simulink library "cables_lib"  (Simulink 7.8)
settings: Solver=ode45  StartTime=0.0  StopTime=10.0  RelTol=1e-3
libraries: powerlib x10
settings Model: Creator=RE25624  LastModifiedBy=g73labuser

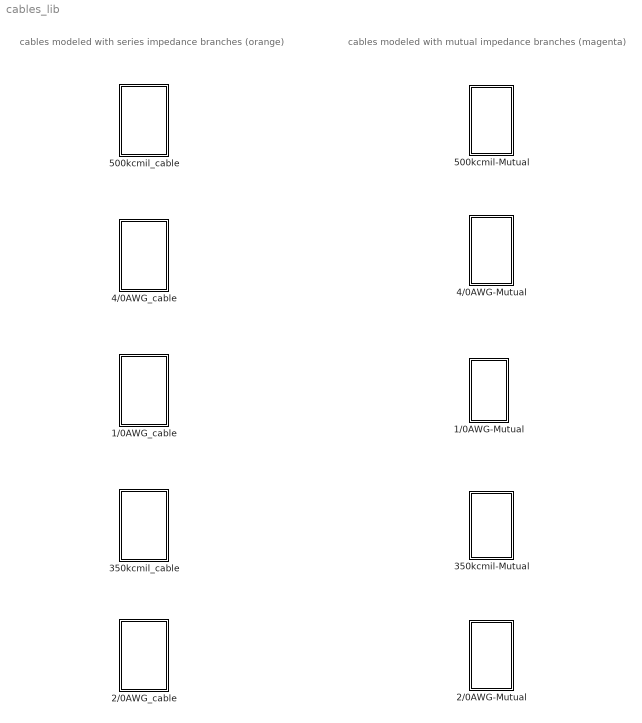
== system cables_lib ==
  note: cables modeled with mutual impedance branches (magenta)
  note: cables modeled with series impedance branches (orange)
  1/0AWG-Mutual : Subsystem  mask(1/0AWG cable){length=1, par_sets=1, ratio=3}
      mask prompts: length "Length [ft]"; par_sets "No. of parallel sets"; ratio "Z0 / Z1 Impedane Ratio"
      mask help:
      | This model approximates a cable using a mutual impedance branch.
      |
      | The parameter values for the positive sequence are based on IEEE 141-1993 Table 4A-7b.
      |
      | The zero-to-positive sequence (Z0/Z1) ratio permits the calculation of the mutual impedance.
      |
      | Example, for a effectively grounded system is in ranges Z0/Z1 < 3.
  1/0AWG_cable : Subsystem  mask(1/0AWG cable){length=50, par_sets=1}
      mask prompts: length "Length [ft]"; par_sets "No. of parallel sets"
      mask help:
      | This block represents a 1/0AWG cable based on Table 4A-7  60 Hz impedance data for three-phase copper cable circuits, in approximate ohms per ft at 75 degrees C (b) Three-conductor cable
      |
      | Page 181 of the Red Book
  2/0AWG-Mutual : Subsystem  mask(2/0AWG cable){length=1, par_sets=1, ratio=3}
      mask prompts: length "Length [ft]"; par_sets "No. of parallel sets"; ratio "Z0 / Z1 Impedane Ratio"
      mask help:
      | This model approximates a cable using a mutual impedance branch.
      |
      | The parameter values for the positive sequence are based on IEEE 141-1993 Table 4A-7b.
      |
      | The zero-to-positive sequence (Z0/Z1) ratio permits the calculation of the mutual impedance.
      |
      | Example, for a effectively grounded system is in ranges Z0/Z1 < 3.
  2/0AWG_cable : Subsystem  mask(2/0AWG cable){length=50, par_sets=1}
      mask prompts: length "Length [ft]"; par_sets "No. of parallel sets"
      mask help:
      | This block represents a 2/0AWG cable based on Table 4A-7  60 Hz impedance data for three-phase copper cable circuits, in approximate ohms per ft at 75 degrees C (b) Three-conductor cable
      |
      | Page 181 of the Red Book
  350kcmil-Mutual : Subsystem  mask(350kcmil cable){length=1, par_sets=1, ratio=3}
      mask prompts: length "Length [ft]"; par_sets "No. of parallel sets"; ratio "Z0 / Z1 Impedane Ratio"
      mask help:
      | This model approximates a cable using a mutual impedance branch.
      |
      | The parameter values for the positive sequence are based on IEEE 141-1993 Table 4A-7b.
      |
      | The zero-to-positive sequence (Z0/Z1) ratio permits the calculation of the mutual impedance.
      |
      | Example, for a effectively grounded system is in ranges Z0/Z1 < 3.
  350kcmil_cable : Subsystem  mask(350kcmil cable){length=50, par_sets=1}
      mask prompts: length "Length [ft]"; par_sets "No. of parallel sets"
      mask help:
      | This block represents a 350kcmil cable based on Table 4A-7  60 Hz impedance data for three-phase copper cable circuits, in approximate ohms per ft at 75 degrees C (b) Three-conductor cable
      |
      | Page 181 of the Red Book
  4/0AWG-Mutual : Subsystem  mask(4/0AWG cable){length=1, par_sets=1, ratio=3}
      mask prompts: length "Length [ft]"; par_sets "No. of parallel sets"; ratio "Z0 / Z1 Impedane Ratio"
      mask help:
      | This model approximates a cable using a mutual impedance branch.
      |
      | The parameter values for the positive sequence are based on IEEE 141-1993 Table 4A-7b.
      |
      | The zero-to-positive sequence (Z0/Z1) ratio permits the calculation of the mutual impedance.
      |
      | Example, for a effectively grounded system is in ranges Z0/Z1 < 3.
  4/0AWG_cable : Subsystem  mask(4/0AWG cable){length=50, par_sets=1}
      mask prompts: length "Length [ft]"; par_sets "No. of parallel sets"
      mask help:
      | This block represents a 4/0AWG cable based on Table 4A-7  60 Hz impedance data for three-phase copper cable circuits, in approximate ohms per ft at 75 degrees C (b) Three-conductor cable
      |
      | Page 181 of the Red Book
  500kcmil-Mutual : Subsystem  mask(500kcmil cable){length=1, par_sets=1, ratio=3}
      mask prompts: length "Length [ft]"; par_sets "No. of parallel sets"; ratio "Z0 / Z1 Impedane Ratio"
      mask help:
      | This model approximates a cable using a mutual impedance branch.
      |
      | The parameter values for the positive sequence are based on IEEE 141-1993 Table 4A-7b.
      |
      | The zero-to-positive sequence (Z0/Z1) ratio permits the calculation of the mutual impedance.
      |
      | Example, for a effectively grounded system is in ranges Z0/Z1 < 3.
  500kcmil_cable : Subsystem  mask(500kcmil cable){length=50, par_sets=1}
      mask prompts: length "Length [ft]"; par_sets "No. of parallel sets"
      mask help:
      | This block represents a 500kcmil cable based on Table 4A-7  60 Hz impedance data for three-phase copper cable circuits, in approximate ohms per ft at 75 degrees C (b) Three-conductor cable
      |
      | Page 181 of the Red Book

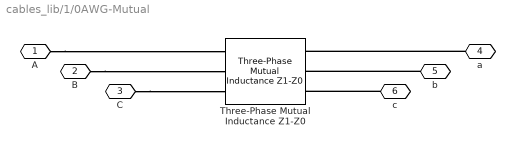
== system cables_lib/1/0AWG-Mutual ==
  Three-Phase Mutual Inductance Z1-Z0 : powerlib/Elements/Three-Phase Mutual Inductance Z1-Z0  LConnTagsString=a|b|c  RConnTagsString=A|B|C  PositiveSequence="[(0.000128*length/par_sets)  (1.0982e-007*length/par_sets)]"  ZeroSequence="[(0.000128*length/par_sets)  (1.0982e-007*length/par_sets)]*ratio"
  A : PMIOPort  Port=1  Side=Left
  B : PMIOPort  Port=2  Side=Left
  C : PMIOPort  Port=3  Side=Left
  a : PMIOPort  Port=4  Side=Right
  b : PMIOPort  Port=5  Side=Right
  c : PMIOPort  Port=6  Side=Right
  connections:
  c/RConn1 -- Three-Phase Mutual Inductance Z1-Z0/RConn3
  C/RConn1 -- Three-Phase Mutual Inductance Z1-Z0/LConn3
  b/RConn1 -- Three-Phase Mutual Inductance Z1-Z0/RConn2
  B/RConn1 -- Three-Phase Mutual Inductance Z1-Z0/LConn2
  a/RConn1 -- Three-Phase Mutual Inductance Z1-Z0/RConn1
  A/RConn1 -- Three-Phase Mutual Inductance Z1-Z0/LConn1

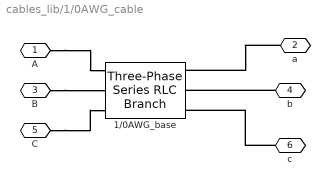
== system cables_lib/1/0AWG_cable ==
  1/0AWG_base : powerlib/Elements/Three-Phase Series RLC Branch  LConnTagsString=A|B|C  RConnTagsString=A|B|C  BranchType=RL  Resistance=0.000128*length/par_sets  Inductance=1.0982e-007*length/par_sets  Capacitance=0  Measurements=None
  A : PMIOPort  Port=1  Side=Left
  a : PMIOPort  Port=2  Side=Right
  B : PMIOPort  Port=3  Side=Left
  b : PMIOPort  Port=4  Side=Right
  C : PMIOPort  Port=5  Side=Left
  c : PMIOPort  Port=6  Side=Right
  connections:
  A/RConn1 -- 1/0AWG_base/LConn1
  a/RConn1 -- 1/0AWG_base/RConn1
  B/RConn1 -- 1/0AWG_base/LConn2
  b/RConn1 -- 1/0AWG_base/RConn2
  C/RConn1 -- 1/0AWG_base/LConn3
  c/RConn1 -- 1/0AWG_base/RConn3

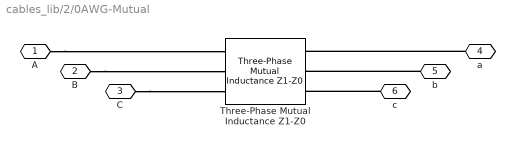
== system cables_lib/2/0AWG-Mutual ==
  Three-Phase Mutual Inductance Z1-Z0 : powerlib/Elements/Three-Phase Mutual Inductance Z1-Z0  LConnTagsString=a|b|c  RConnTagsString=A|B|C  PositiveSequence="[(0.000102*length/par_sets)  (1.0796e-007*length/par_sets)]"  ZeroSequence="[(0.000102*length/par_sets)  (1.0796e-007*length/par_sets)]*ratio"
  A : PMIOPort  Port=1  Side=Left
  B : PMIOPort  Port=2  Side=Left
  C : PMIOPort  Port=3  Side=Left
  a : PMIOPort  Port=4  Side=Right
  b : PMIOPort  Port=5  Side=Right
  c : PMIOPort  Port=6  Side=Right
  connections:
  c/RConn1 -- Three-Phase Mutual Inductance Z1-Z0/RConn3
  C/RConn1 -- Three-Phase Mutual Inductance Z1-Z0/LConn3
  b/RConn1 -- Three-Phase Mutual Inductance Z1-Z0/RConn2
  B/RConn1 -- Three-Phase Mutual Inductance Z1-Z0/LConn2
  a/RConn1 -- Three-Phase Mutual Inductance Z1-Z0/RConn1
  A/RConn1 -- Three-Phase Mutual Inductance Z1-Z0/LConn1

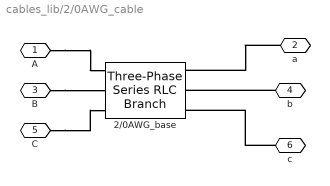
== system cables_lib/2/0AWG_cable ==
  2/0AWG_base : powerlib/Elements/Three-Phase Series RLC Branch  LConnTagsString=A|B|C  RConnTagsString=A|B|C  BranchType=RL  Resistance=0.000102*length/par_sets  Inductance=1.0796e-007*length/par_sets  Capacitance=0  Measurements=None
  A : PMIOPort  Port=1  Side=Left
  a : PMIOPort  Port=2  Side=Right
  B : PMIOPort  Port=3  Side=Left
  b : PMIOPort  Port=4  Side=Right
  C : PMIOPort  Port=5  Side=Left
  c : PMIOPort  Port=6  Side=Right
  connections:
  A/RConn1 -- 2/0AWG_base/LConn1
  a/RConn1 -- 2/0AWG_base/RConn1
  B/RConn1 -- 2/0AWG_base/LConn2
  b/RConn1 -- 2/0AWG_base/RConn2
  C/RConn1 -- 2/0AWG_base/LConn3
  c/RConn1 -- 2/0AWG_base/RConn3

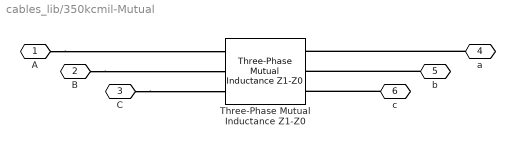
== system cables_lib/350kcmil-Mutual ==
  Three-Phase Mutual Inductance Z1-Z0 : powerlib/Elements/Three-Phase Mutual Inductance Z1-Z0  LConnTagsString=a|b|c  RConnTagsString=A|B|C  PositiveSequence="[(3.78e-005*length/par_sets)  (9.8941e-008*length/par_sets)]"  ZeroSequence="[(3.78e-005*length/par_sets)  (9.8941e-008*length/par_sets)]*ratio"
  A : PMIOPort  Port=1  Side=Left
  B : PMIOPort  Port=2  Side=Left
  C : PMIOPort  Port=3  Side=Left
  a : PMIOPort  Port=4  Side=Right
  b : PMIOPort  Port=5  Side=Right
  c : PMIOPort  Port=6  Side=Right
  connections:
  c/RConn1 -- Three-Phase Mutual Inductance Z1-Z0/RConn3
  C/RConn1 -- Three-Phase Mutual Inductance Z1-Z0/LConn3
  b/RConn1 -- Three-Phase Mutual Inductance Z1-Z0/RConn2
  B/RConn1 -- Three-Phase Mutual Inductance Z1-Z0/LConn2
  a/RConn1 -- Three-Phase Mutual Inductance Z1-Z0/RConn1
  A/RConn1 -- Three-Phase Mutual Inductance Z1-Z0/LConn1

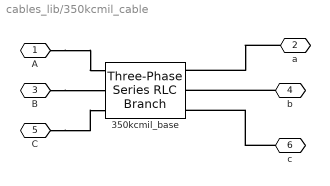
== system cables_lib/350kcmil_cable ==
  350kcmil_base : powerlib/Elements/Three-Phase Series RLC Branch  LConnTagsString=A|B|C  RConnTagsString=A|B|C  BranchType=RL  Resistance=3.78e-005*length/par_sets  Inductance=9.8941e-008*length/par_sets  Capacitance=0  Measurements=None
  A : PMIOPort  Port=1  Side=Left
  a : PMIOPort  Port=2  Side=Right
  B : PMIOPort  Port=3  Side=Left
  b : PMIOPort  Port=4  Side=Right
  C : PMIOPort  Port=5  Side=Left
  c : PMIOPort  Port=6  Side=Right
  connections:
  A/RConn1 -- 350kcmil_base/LConn1
  a/RConn1 -- 350kcmil_base/RConn1
  B/RConn1 -- 350kcmil_base/LConn2
  b/RConn1 -- 350kcmil_base/RConn2
  C/RConn1 -- 350kcmil_base/LConn3
  c/RConn1 -- 350kcmil_base/RConn3

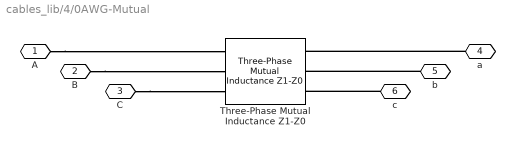
== system cables_lib/4/0AWG-Mutual ==
  Three-Phase Mutual Inductance Z1-Z0 : powerlib/Elements/Three-Phase Mutual Inductance Z1-Z0  LConnTagsString=a|b|c  RConnTagsString=A|B|C  PositiveSequence="[(6.4e-005*length/par_sets)  (1.0106e-007*length/par_sets)]"  ZeroSequence="[(6.4e-005*length/par_sets)  (1.0106e-007*length/par_sets)]*ratio"
  A : PMIOPort  Port=1  Side=Left
  B : PMIOPort  Port=2  Side=Left
  C : PMIOPort  Port=3  Side=Left
  a : PMIOPort  Port=4  Side=Right
  b : PMIOPort  Port=5  Side=Right
  c : PMIOPort  Port=6  Side=Right
  connections:
  c/RConn1 -- Three-Phase Mutual Inductance Z1-Z0/RConn3
  C/RConn1 -- Three-Phase Mutual Inductance Z1-Z0/LConn3
  b/RConn1 -- Three-Phase Mutual Inductance Z1-Z0/RConn2
  B/RConn1 -- Three-Phase Mutual Inductance Z1-Z0/LConn2
  a/RConn1 -- Three-Phase Mutual Inductance Z1-Z0/RConn1
  A/RConn1 -- Three-Phase Mutual Inductance Z1-Z0/LConn1

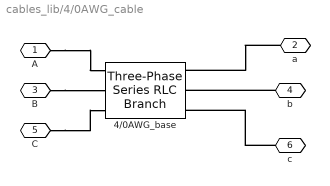
== system cables_lib/4/0AWG_cable ==
  4/0AWG_base : powerlib/Elements/Three-Phase Series RLC Branch  LConnTagsString=A|B|C  RConnTagsString=A|B|C  BranchType=RL  Resistance=6.4e-005*length/par_sets  Inductance=1.0106e-007*length/par_sets  Capacitance=0  Measurements=None
  A : PMIOPort  Port=1  Side=Left
  a : PMIOPort  Port=2  Side=Right
  B : PMIOPort  Port=3  Side=Left
  b : PMIOPort  Port=4  Side=Right
  C : PMIOPort  Port=5  Side=Left
  c : PMIOPort  Port=6  Side=Right
  connections:
  A/RConn1 -- 4/0AWG_base/LConn1
  a/RConn1 -- 4/0AWG_base/RConn1
  B/RConn1 -- 4/0AWG_base/LConn2
  b/RConn1 -- 4/0AWG_base/RConn2
  C/RConn1 -- 4/0AWG_base/LConn3
  c/RConn1 -- 4/0AWG_base/RConn3

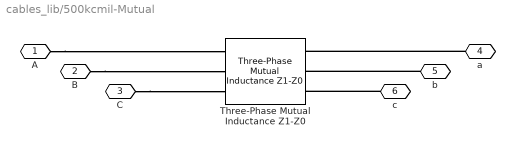
== system cables_lib/500kcmil-Mutual ==
  Three-Phase Mutual Inductance Z1-Z0 : powerlib/Elements/Three-Phase Mutual Inductance Z1-Z0  LConnTagsString=a|b|c  RConnTagsString=A|B|C  PositiveSequence="[(2.94e-005*length/par_sets)  (9.2575e-008*length/par_sets)]"  ZeroSequence="[(2.94e-005*length/par_sets)  (9.2575e-008*length/par_sets)]*ratio"
  A : PMIOPort  Port=1  Side=Left
  B : PMIOPort  Port=2  Side=Left
  C : PMIOPort  Port=3  Side=Left
  a : PMIOPort  Port=4  Side=Right
  b : PMIOPort  Port=5  Side=Right
  c : PMIOPort  Port=6  Side=Right
  connections:
  c/RConn1 -- Three-Phase Mutual Inductance Z1-Z0/RConn3
  C/RConn1 -- Three-Phase Mutual Inductance Z1-Z0/LConn3
  b/RConn1 -- Three-Phase Mutual Inductance Z1-Z0/RConn2
  B/RConn1 -- Three-Phase Mutual Inductance Z1-Z0/LConn2
  a/RConn1 -- Three-Phase Mutual Inductance Z1-Z0/RConn1
  A/RConn1 -- Three-Phase Mutual Inductance Z1-Z0/LConn1

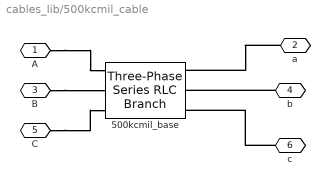
== system cables_lib/500kcmil_cable ==
  500kcmil_base : powerlib/Elements/Three-Phase Series RLC Branch  LConnTagsString=A|B|C  RConnTagsString=A|B|C  BranchType=RL  Resistance=2.94e-005*length/par_sets  Inductance=9.2575e-008*length/par_sets  Capacitance=0  Measurements=None
  A : PMIOPort  Port=1  Side=Left
  a : PMIOPort  Port=2  Side=Right
  B : PMIOPort  Port=3  Side=Left
  b : PMIOPort  Port=4  Side=Right
  C : PMIOPort  Port=5  Side=Left
  c : PMIOPort  Port=6  Side=Right
  connections:
  A/RConn1 -- 500kcmil_base/LConn1
  a/RConn1 -- 500kcmil_base/RConn1
  B/RConn1 -- 500kcmil_base/LConn2
  b/RConn1 -- 500kcmil_base/RConn2
  C/RConn1 -- 500kcmil_base/LConn3
  c/RConn1 -- 500kcmil_base/RConn3
